simulink model "qcar_sensor_validation"  (R2024b)
settings: Solver=ode1  StartTime=0.0  StopTime=inf  FixedStep=Controller_Sample_Time  RelTol=1e-3  EnableMultiTasking=on
undefined symbols (not defined in the file): AAAF5050, angles_qcar2, cal_pos, Controller_Sample_Time, CSI_Sample_Time, gcbh, GyroKF_P0, GyroKF_Q, GyroKF_R, GyroKF_X0, height, HIL, ImageDisplay_Sample_Time, Initialization_Time, JPEG, K12, left, LiDAR_Sample_Time, MC, path_x4, path_y4, Point, qc_get_step_size, qcar2_lidar_to_body_rotation, qcar2_lidar_to_map_rotation, qcar2_virtual_to_physical_lidar_rotation, QCarEKF_L, QCarEKF_P0, QCarEKF_Q, QCarEKF_R_combined, QCarEKF_R_heading, QcarKF_X0, range_qcar2, RealSense_Sample_Time, steering_Kd, steering_Kp, top, video_display_show, width
libraries: quarc_library x45, simulink_extras x6, simulink x3, mspfiltlib x1
(part 2 of 3)

== system qcar_sensor_validation/writeToQCarDAC ==
  note: 11: LED left outside brake light
      | 12: LED left inside brake light
      | 12: LED right inside brake light
      | 13: LED right outside brake fight
      | 14: LED left reverse light
      | 15: LED right reverse light
      | 16: LED left rear signal
      | 17: LED right rear signal
      | 18: LED left outside headlight
      | 19: LED left middle headlight
      | 20: LED left inside headlight
      | 21: LED right inside headlight
      | 22: LED right middle headlight
      | 23: LED right outside headlight
      | 24: LED left front signal
      | 25: LED right front signal
  motor_cmd [1] (%) : Inport
  steering_cmd [1] (rad) : Inport  Port=2
  leds [14] (bool) : Inport  Port=3
  ledStrip [R,G,B] (%) : Inport  Port=4
  Gain : Gain
  HIL Write : quarc_library/Data Acquisition/Generic/Immediate I//O/HIL Write  object_name=HIL-2  analog_channels=[]  pwm_channels=[]  digital_channels=[11:26]  other_channels=[1000 11000]  sample_time=-1  active=on  vector_input=on
  LED Strip : quarc_library/Devices/Third-Party/Displays/LED Strip  led_type=AAAF5050-MC-K12  uri=tcpip://localhost:18969  mode=uniform  max_leds=33  initial_red=[0.000]  initial_green=[1.000]  initial_blue=[0.000]  final_red=[0]  final_green=[0]  final_blue=[0]  sample_time=ImageDisplay_Sample_Time  use_vectors=off  active=off
      settings: SourceProductName=QUARC Targets
  Mux : Mux  Inputs=2
  Steering Bias : Bias  Bias=-0.05  SaturateOnIntegerOverflow=off
  Terminator : Terminator
  motor sat : Saturate  UpperLimit=.6  LowerLimit=-0.6
  steering sat : Saturate
  wires:
  ledStrip [R,G,B] (%)/1 -> LED Strip/1
  steering_cmd [1] (rad)/1 -> Steering Bias/1
  motor sat/1 -> Mux/2
  steering sat/1 -> Mux/1
  leds [14] (bool)/1 -> HIL Write/1
  Steering Bias/1 -> Gain/1
  motor_cmd [1] (%)/1 -> motor sat/1
  LED Strip/1 -> Terminator/1
  Gain/1 -> steering sat/1
  Mux/1 -> HIL Write/2

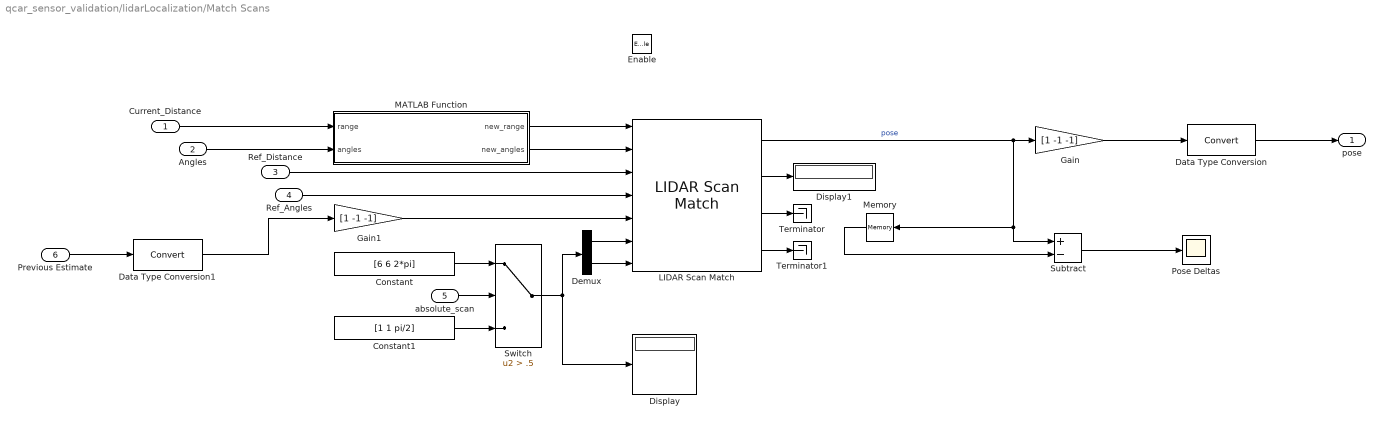
== system qcar_sensor_validation/lidarLocalization/Match Scans ==
  Current_Distance : Inport
  Angles : Inport  Port=2
  Ref_Distance : Inport  Port=3
  Ref_Angles : Inport  Port=4
  absolute_scan : Inport  Port=5
  Previous Estimate : Inport  Port=6
  Enable : EnablePort  PropagateVarSize=During execution
  Constant : Constant  Value=[6 6 2*pi]
  Constant1 : Constant  Value=[1 1 pi/2]
  Data Type Conversion : DataTypeConversion  SaturateOnIntegerOverflow=off  RndMeth=Floor
  Data Type Conversion1 : DataTypeConversion  SaturateOnIntegerOverflow=off  RndMeth=Floor
  Demux : Demux  Outputs=2
  Display : Display
  Display1 : Display
  Gain : Gain  Gain=[1 -1 -1]
  Gain1 : Gain  Gain=[1 -1 -1]
  LIDAR Scan Match : quarc_library/Image Processing/Generic/LIDAR Scan Match  mode=Variable-size input  resolution=35  max_range=8  use_initial_pose=on
      settings: SourceProductName=QUARC Targets
  MATLAB Function : MATLAB Function  TreatAsAtomicUnit=on
  Memory : Memory  InitialCondition=[0 0 0]  InheritSampleTime=on  LinearizeMemory=on  LinearizeAsDelay=on
  Pose Deltas : Scope
  Subtract : Sum  Inputs=+-
  Switch : Switch  Criteria=u2 > Threshold  Threshold=.5  SaturateOnIntegerOverflow=off  InputSameDT=off
  Terminator : Terminator
  Terminator1 : Terminator
  pose : Outport
  wires:
  LIDAR Scan Match/1 -> Subtract/1, Memory/1, Gain/1  "pose"
  Ref_Distance/1 -> LIDAR Scan Match/3
  Ref_Angles/1 -> LIDAR Scan Match/4
  Gain/1 -> Data Type Conversion/1
  Memory/1 -> Subtract/2
  absolute_scan/1 -> Switch/2
  Switch/1 -> Demux/1, Display/1
  Demux/1 -> LIDAR Scan Match/6
  Demux/2 -> LIDAR Scan Match/7
  Constant/1 -> Switch/1
  Constant1/1 -> Switch/3
  Data Type Conversion/1 -> pose/1
  MATLAB Function/1(new_range) -> LIDAR Scan Match/1
  MATLAB Function/2(new_angles) -> LIDAR Scan Match/2
  Subtract/1 -> Pose Deltas/1
  Previous Estimate/1 -> Data Type Conversion1/1
  Gain1/1 -> LIDAR Scan Match/5
  Data Type Conversion1/1 -> Gain1/1
  Current_Distance/1 -> MATLAB Function/1(range)
  Angles/1 -> MATLAB Function/2(angles)
  LIDAR Scan Match/3 -> Terminator/1
  LIDAR Scan Match/4 -> Terminator1/1
  LIDAR Scan Match/2 -> Display1/1

== system qcar_sensor_validation/lidarLocalization/RisingEdge ==
  Input : Inport
  Logical Operator1 : Logic  AllPortsSameDT=off
  Logical Operator2 : Logic  Operator=NOT  AllPortsSameDT=off
  Memory : Memory  InheritSampleTime=on  LinearizeMemory=on
  RisingEdgeTrigger : Outport  VectorParamsAs1DForOutWhenUnconnected=off
  wires:
  Logical Operator1/1 -> RisingEdgeTrigger/1
  Logical Operator2/1 -> Logical Operator1/2
  Memory/1 -> Logical Operator2/1
  Input/1 -> Logical Operator1/1, Memory/1

== system qcar_sensor_validation/lidarLocalization/rising edge latch ==
  rising edge trigger : Inport
  input : Inport  Port=2
  untriggered output : Inport  Port=3
  Latch Input : Subsystem  TreatAsAtomicUnit=on
  Switch : Switch  Threshold=0.5  SaturateOnIntegerOverflow=off  InputSameDT=off
  output : Outport  VectorParamsAs1DForOutWhenUnconnected=off
  wires:
  untriggered output/1 -> Switch/3
  Switch/1 -> output/1
  Latch Input/1(Latch) -> Switch/1
  Latch Input/2(Executed) -> Switch/2
  input/1 -> Latch Input/1(Input)
  rising edge trigger/1 -> Latch Input/Trigger

== system qcar_sensor_validation/obstacleDetection/Newer Depth ==
  In1 : Inport
  Channel : quarc_library/Signal Routing/Channel  channel=0  buffer_size=1
  Image Compress : quarc_library/Image Processing/Generic/Image Compress  algorithm=JPEG  source=Internal dialog parameter  quality=quality  output_dim=-1
  Video Display : quarc_library/Multimedia/Video Display  Tag=qcar_sensor_validation/obstacleDetection/Newer Depth/Video Display  sample_time=sample_time  use_hardware=on
  wires:
  Image Compress/1 -> Channel/1
  In1/1 -> Image Compress/1
  Channel/1 -> Video Display/1

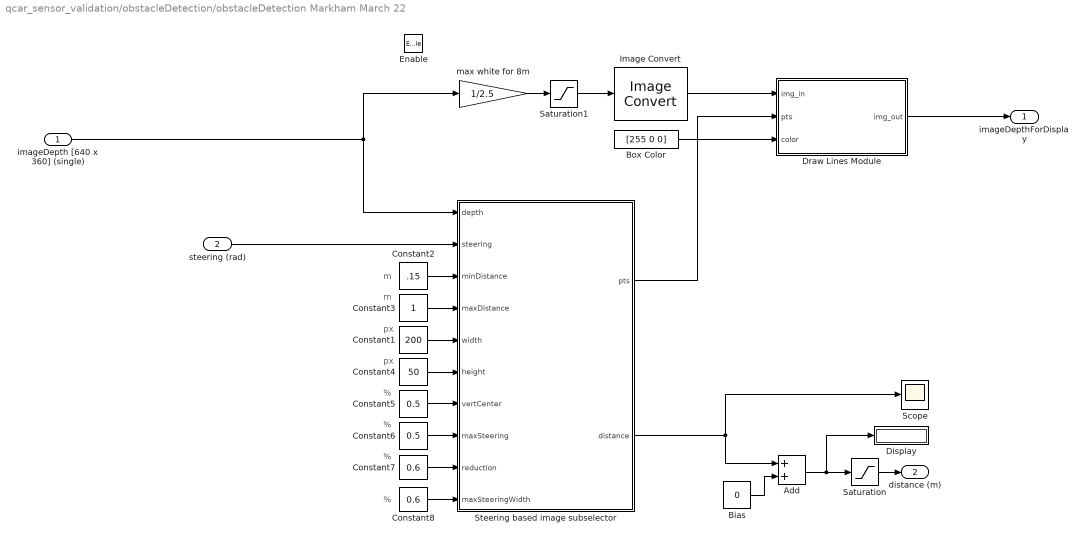
== system qcar_sensor_validation/obstacleDetection/obstacleDetection Markham March 22 ==
  note: %
  note: m
  note: m
  note: %
  note: px
  note: px
  note: %
  note: %
  imageDepth [640 x 360] (single) : Inport
  steering (rad) : Inport  Port=2
  Enable : EnablePort  PropagateVarSize=During execution
  Add : Sum
  Bias : Constant  Value=0
  Box Color : Constant  Value=[255 0 0]
  Constant1 : Constant  Value=200
  Constant2 : Constant  Value=.15
  Constant3 : Constant
  Constant4 : Constant  Value=50
  Constant5 : Constant  Value=0.5
  Constant6 : Constant  Value=0.5
  Constant7 : Constant  Value=0.6
  Constant8 : Constant  Value=0.6
  Display : Display
  Draw Lines Module : MATLAB Function  TreatAsAtomicUnit=on
  Image Convert : quarc_library/Image Processing/Generic/Image Convert  input_format=MATLAB greyscale (HxW)  padding=0  output_format=MATLAB greyscale (HxW)  data_type=uint16
      settings: AttributesFormatString=(%<input_format>)  SourceProductName=QUARC Targets
  Saturation : Saturate  UpperLimit=2  LowerLimit=0.05
  Saturation1 : Saturate  UpperLimit=1  LowerLimit=0
  Scope : Scope
  Steering based image subselector : MATLAB Function  TreatAsAtomicUnit=on
  max white for 8m : Gain  Gain=1/2.5
  imageDepthForDisplay : Outport  VectorParamsAs1DForOutWhenUnconnected=off
  distance (m) : Outport  Port=2  VectorParamsAs1DForOutWhenUnconnected=off
  wires:
  Saturation1/1 -> Image Convert/1
  Constant6/1 -> Steering based image subselector/8(maxSteering)
  Steering based image subselector/2(distance) -> Add/1, Scope/1
  Constant5/1 -> Steering based image subselector/7(vertCenter)
  Constant4/1 -> Steering based image subselector/6(height)
  Constant1/1 -> Steering based image subselector/5(width)
  Constant3/1 -> Steering based image subselector/4(maxDistance)
  Constant2/1 -> Steering based image subselector/3(minDistance)
  steering (rad)/1 -> Steering based image subselector/2(steering)
  Draw Lines Module/1(img_out) -> imageDepthForDisplay/1
  Steering based image subselector/1(pts) -> Draw Lines Module/2(pts)
  Image Convert/1 -> Draw Lines Module/1(img_in)
  max white for 8m/1 -> Saturation1/1
  imageDepth [640 x 360] (single)/1 -> Steering based image subselector/1(depth), max white for 8m/1
  Bias/1 -> Add/2
  Add/1 -> Saturation/1, Display/1
  Saturation/1 -> distance (m)/1
  Box Color/1 -> Draw Lines Module/3(color)
  Constant7/1 -> Steering based image subselector/9(reduction)
  Constant8/1 -> Steering based image subselector/10(maxSteeringWidth)

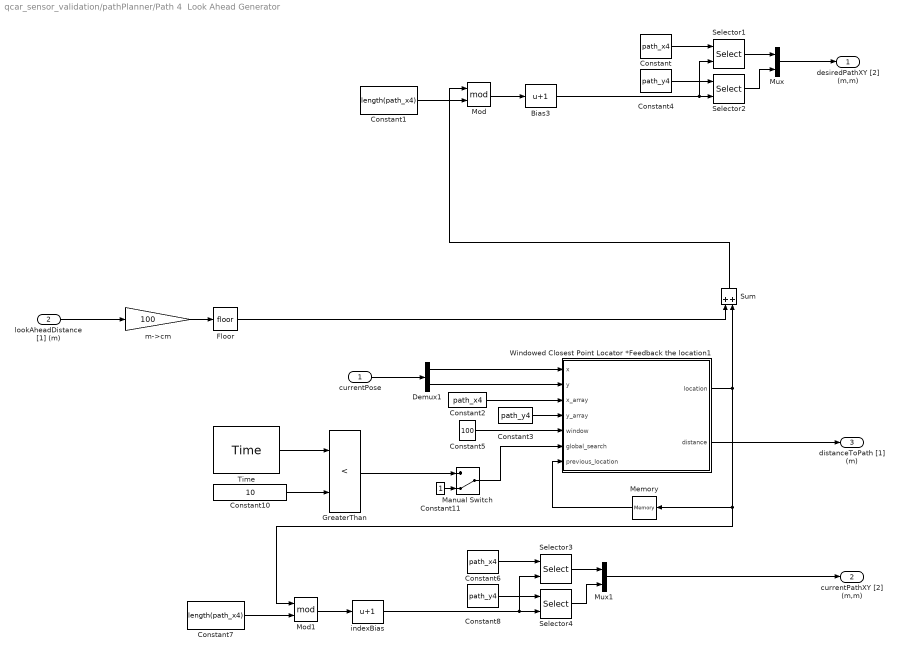
== system qcar_sensor_validation/pathPlanner/Path 4  Look Ahead Generator ==
  currentPose : Inport
  lookAheadDistance [1] (m) : Inport  Port=2
  Bias3 : Bias  Bias=1  SaturateOnIntegerOverflow=off
  Constant : Constant  Value=path_x4
  Constant1 : Constant  Value=length(path_x4)
  Constant10 : Constant  Value=10
  Constant11 : Constant
  Constant2 : Constant  Value=path_x4
  Constant3 : Constant  Value=path_y4
  Constant4 : Constant  Value=path_y4
  Constant5 : Constant  Value=100
  Constant6 : Constant  Value=path_x4
  Constant7 : Constant  Value=length(path_x4)
  Constant8 : Constant  Value=path_y4
  Demux1 : Demux  Outputs=2
  Floor : Rounding
  GreaterThan : RelationalOperator  Operator=<  OutDataTypeStr=boolean  RndMeth=Simplest  InputSameDT=off
  Manual Switch : ManualSwitch  CurrentSetting=0
  Memory : Memory  InitialCondition=1  InheritSampleTime=on  LinearizeMemory=on  LinearizeAsDelay=on
  Mod : Math  Operator=mod
  Mod1 : Math  Operator=mod
  Mux : Mux  Inputs=2
  Mux1 : Mux  Inputs=2
  Selector{1..4} (4 alike) : Selector  InputPortWidth=length(path_x4)  IndexOptions=Index vector (port)  Indices=[1 3]  OutputSizes=1
  Sum : Sum
  Time : quarc_library/Sources/Time/Time  time_source=Wall clock  sample_time=qc_get_step_size
  Windowed Closest Point Locator *Feedback the location1 : MATLAB Function  TreatAsAtomicUnit=on
  indexBias : Bias  Bias=1  SaturateOnIntegerOverflow=off
  m->cm : Gain  Gain=100
  desiredPathXY [2] (m,m) : Outport
  currentPathXY [2] (m,m) : Outport  Port=2
  distanceToPath [1] (m) : Outport  Port=3
  wires:
  Windowed Closest Point Locator *Feedback the location1/1(location) -> Mod1/1, Memory/1, Sum/2
  Memory/1 -> Windowed Closest Point Locator *Feedback the location1/7(previous_location)
  Constant5/1 -> Windowed Closest Point Locator *Feedback the location1/5(window)
  Bias3/1 -> Selector2/2, Selector1/2
  Windowed Closest Point Locator *Feedback the location1/2(distance) -> distanceToPath [1] (m)/1
  Selector2/1 -> Mux/2
  Mux/1 -> desiredPathXY [2] (m,m)/1
  Constant4/1 -> Selector2/1
  Selector1/1 -> Mux/1
  Constant/1 -> Selector1/1
  Floor/1 -> Sum/1
  m->cm/1 -> Floor/1
  lookAheadDistance [1] (m)/1 -> m->cm/1
  currentPose/1 -> Demux1/1
  Mod/1 -> Bias3/1
  Demux1/2 -> Windowed Closest Point Locator *Feedback the location1/2(y)
  Sum/1 -> Mod/1
  Constant1/1 -> Mod/2
  Constant3/1 -> Windowed Closest Point Locator *Feedback the location1/4(y_array)
  Constant2/1 -> Windowed Closest Point Locator *Feedback the location1/3(x_array)
  Demux1/1 -> Windowed Closest Point Locator *Feedback the location1/1(x)
  Mux1/1 -> currentPathXY [2] (m,m)/1
  Mod1/1 -> indexBias/1
  Selector4/1 -> Mux1/2
  Constant7/1 -> Mod1/2
  Selector3/1 -> Mux1/1
  Constant8/1 -> Selector4/1
  indexBias/1 -> Selector3/2, Selector4/2
  Constant6/1 -> Selector3/1
  Time/1 -> GreaterThan/1
  Constant10/1 -> GreaterThan/2
  Manual Switch/1 -> Windowed Closest Point Locator *Feedback the location1/6(global_search)
  Constant11/1 -> Manual Switch/2
  GreaterThan/1 -> Manual Switch/1

== system qcar_sensor_validation/pathPlanner/rateAligner ==
  xy 1 : Inport
  xy 2 : Inport  Port=2
  Demux1 : Demux  Outputs=2
  Demux2 : Demux  Outputs=2
  Mux : Mux  Inputs=2
  Mux1 : Mux  Inputs=2
  Rate Transition1 : RateTransition  OutPortSampleTime=ImageDisplay_Sample_Time
  Rate Transition2 : RateTransition  OutPortSampleTime=ImageDisplay_Sample_Time
  x : Outport
  y : Outport  Port=2
  wires:
  Demux2/1 -> Mux/2
  Demux1/2 -> Mux1/1
  Demux1/1 -> Mux/1
  Demux2/2 -> Mux1/2
  Mux/1 -> x/1
  Mux1/1 -> y/1
  xy 1/1 -> Rate Transition1/1
  Rate Transition1/1 -> Demux1/1
  xy 2/1 -> Rate Transition2/1
  Rate Transition2/1 -> Demux2/1

== system qcar_sensor_validation/rateTimingPlots/monitorTiming ==
  note: Timing Performance
  note: moniorTiming Module:
      |
      | This subsystem outputs the sample time and computation time of the model.
      |
      | Outputs:
      | sampleTime (s) n/a : Sample time (unfiltered and filtered) in seconds.
      | computationTime (s) n/a : Computation time (unfiltered and filtered) in seconds.
      |
      | Usage:
      | Compare the Sample Time (s) output to a constant (qc_get_step_size) to monitor whether or not the desired sample time is being achieved. The Computation Time (s) values should be lower than the corresponding sample time value to ensure that the solver has enough time per time step.
  Computation Time : quarc_library/Sources/Time/Computation Time  sample_time=CSI_Sample_Time  use_model=on  use_cpu_time=off
  Constant : Constant  Value=CSI_Sample_Time  SampleTime=-1
  Mux : Mux  Inputs=3
  Sample Time : quarc_library/Sources/Time/Sample Time  Priority=-99  sample_time=CSI_Sample_Time
  Timing (s) : Outport  VectorParamsAs1DForOutWhenUnconnected=off
  wires:
  Computation Time/1 -> Mux/3
  Mux/1 -> Timing (s)/1
  Sample Time/1 -> Mux/1
  Constant/1 -> Mux/2

== system qcar_sensor_validation/rateTimingPlots/monitorTiming1 ==
  note: moniorTiming Module:
      |
      | This subsystem outputs the sample time and computation time of the model.
      |
      | Outputs:
      | sampleTime (s) n/a : Sample time (unfiltered and filtered) in seconds.
      | computationTime (s) n/a : Computation time (unfiltered and filtered) in seconds.
      |
      | Usage:
      | Compare the Sample Time (s) output to a constant (qc_get_step_size) to monitor whether or not the desired sample time is being achieved. The Computation Time (s) values should be lower than the corresponding sample time value to ensure that the solver has enough time per time step.
  note: Timing Performance
  Computation Time : quarc_library/Sources/Time/Computation Time  sample_time=qc_get_step_size  use_model=on  use_cpu_time=off
  Constant : Constant  Value=qc_get_step_size  SampleTime=-1
  Mux : Mux  Inputs=3
  Sample Time : quarc_library/Sources/Time/Sample Time  Priority=-99  sample_time=qc_get_step_size
  Timing (s) : Outport  VectorParamsAs1DForOutWhenUnconnected=off
  wires:
  Constant/1 -> Mux/2
  Sample Time/1 -> Mux/1
  Mux/1 -> Timing (s)/1
  Computation Time/1 -> Mux/3

== system qcar_sensor_validation/rateTimingPlots/monitorTiming2 ==
  note: moniorTiming Module:
      |
      | This subsystem outputs the sample time and computation time of the model.
      |
      | Outputs:
      | sampleTime (s) n/a : Sample time (unfiltered and filtered) in seconds.
      | computationTime (s) n/a : Computation time (unfiltered and filtered) in seconds.
      |
      | Usage:
      | Compare the Sample Time (s) output to a constant (qc_get_step_size) to monitor whether or not the desired sample time is being achieved. The Computation Time (s) values should be lower than the corresponding sample time value to ensure that the solver has enough time per time step.
  note: Timing Performance
  Computation Time : quarc_library/Sources/Time/Computation Time  sample_time=RealSense_Sample_Time  use_model=on  use_cpu_time=off
  Constant : Constant  Value=RealSense_Sample_Time  SampleTime=-1
  Mux : Mux  Inputs=3
  Sample Time : quarc_library/Sources/Time/Sample Time  Priority=-99  sample_time=RealSense_Sample_Time
  Timing (s) : Outport  VectorParamsAs1DForOutWhenUnconnected=off
  wires:
  Constant/1 -> Mux/2
  Sample Time/1 -> Mux/1
  Mux/1 -> Timing (s)/1
  Computation Time/1 -> Mux/3

== system qcar_sensor_validation/rateTimingPlots/monitorTiming3 ==
  note: Timing Performance
  note: moniorTiming Module:
      |
      | This subsystem outputs the sample time and computation time of the model.
      |
      | Outputs:
      | sampleTime (s) n/a : Sample time (unfiltered and filtered) in seconds.
      | computationTime (s) n/a : Computation time (unfiltered and filtered) in seconds.
      |
      | Usage:
      | Compare the Sample Time (s) output to a constant (qc_get_step_size) to monitor whether or not the desired sample time is being achieved. The Computation Time (s) values should be lower than the corresponding sample time value to ensure that the solver has enough time per time step.
  Computation Time : quarc_library/Sources/Time/Computation Time  sample_time=ImageDisplay_Sample_Time  use_model=on  use_cpu_time=off
  Constant : Constant  Value=ImageDisplay_Sample_Time  SampleTime=-1
  Mux : Mux  Inputs=3
  Sample Time : quarc_library/Sources/Time/Sample Time  Priority=-99  sample_time=ImageDisplay_Sample_Time
  Timing (s) : Outport  VectorParamsAs1DForOutWhenUnconnected=off
  wires:
  Computation Time/1 -> Mux/3
  Mux/1 -> Timing (s)/1
  Sample Time/1 -> Mux/1
  Constant/1 -> Mux/2

== system qcar_sensor_validation/rateTimingPlots/monitorTiming5 ==
  note: moniorTiming Module:
      |
      | This subsystem outputs the sample time and computation time of the model.
      |
      | Outputs:
      | sampleTime (s) n/a : Sample time (unfiltered and filtered) in seconds.
      | computationTime (s) n/a : Computation time (unfiltered and filtered) in seconds.
      |
      | Usage:
      | Compare the Sample Time (s) output to a constant (qc_get_step_size) to monitor whether or not the desired sample time is being achieved. The Computation Time (s) values should be lower than the corresponding sample time value to ensure that the solver has enough time per time step.
  note: Timing Performance
  Computation Time : quarc_library/Sources/Time/Computation Time  sample_time=LiDAR_Sample_Time  use_model=on  use_cpu_time=off
  Constant : Constant  Value=LiDAR_Sample_Time  SampleTime=-1
  Mux : Mux  Inputs=3
  Sample Time : quarc_library/Sources/Time/Sample Time  Priority=-99  sample_time=LiDAR_Sample_Time
  Timing (s) : Outport  VectorParamsAs1DForOutWhenUnconnected=off
  wires:
  Constant/1 -> Mux/2
  Sample Time/1 -> Mux/1
  Mux/1 -> Timing (s)/1
  Computation Time/1 -> Mux/3

== system qcar_sensor_validation/rateTimingPlots/monitorTiming7 ==
  note: Timing Performance
  note: moniorTiming Module:
      |
      | This subsystem outputs the sample time and computation time of the model.
      |
      | Outputs:
      | sampleTime (s) n/a : Sample time (unfiltered and filtered) in seconds.
      | computationTime (s) n/a : Computation time (unfiltered and filtered) in seconds.
      |
      | Usage:
      | Compare the Sample Time (s) output to a constant (qc_get_step_size) to monitor whether or not the desired sample time is being achieved. The Computation Time (s) values should be lower than the corresponding sample time value to ensure that the solver has enough time per time step.
  Computation Time : quarc_library/Sources/Time/Computation Time  sample_time=1  use_model=on  use_cpu_time=off
  Constant : Constant  SampleTime=-1
  Mux : Mux  Inputs=3
  Sample Time : quarc_library/Sources/Time/Sample Time  Priority=-99  sample_time=1
  Timing (s) : Outport  VectorParamsAs1DForOutWhenUnconnected=off
  wires:
  Computation Time/1 -> Mux/3
  Mux/1 -> Timing (s)/1
  Sample Time/1 -> Mux/1
  Constant/1 -> Mux/2

== system qcar_sensor_validation/readQCarDAC/counts to meters ==
  note: Estimate car speed from motor encoder counts rate
  note: v = 2*pi*r * omega (if omega is in rot/s)
      | v = r * omega (if omega is in rad/s)
      | r = 0.0342 m
  note: (Diff. pinion*pinion)/(Spur*Diff. spur)
  note: speedEstimation Module:
      |
      | This subsystem converts the motor speed measurements in counts/s to a useful longitudinal car speed in m/s.
      |
      | Inputs:
      | motorSpeed (counts/s) n/a : Drive motor speed measured using an encoder
      |
      | Outputs:
      | longitudinalCarSpeed (m/s) n/a : The platform's longitudinal speed (along the front-rear axis direction)
  motorSpeed (counts/s) : Inport
  counts to rotations : Gain  Gain=1/720/4
  gear ratios : Gain  Gain=(13*19)/(70*37)
  rot/s to rad/s : Gain  Gain=2*pi
  wheel radius : Gain  Gain=0.0342
  longitudinalCarSpeed (m/s) : Outport  VectorParamsAs1DForOutWhenUnconnected=off
  wires:
  motorSpeed (counts/s)/1 -> counts to rotations/1
  rot/s to rad/s/1 -> wheel radius/1  "wheel speed (rad/s)"
  counts to rotations/1 -> gear ratios/1  "motor speed (rot/s)"
  wheel radius/1 -> longitudinalCarSpeed (m/s)/1  "wheel speed (m/s)"
  gear ratios/1 -> rot/s to rad/s/1  "shaft speed (rots/s)"

== system qcar_sensor_validation/readQCarDAC/counts//s to m//s ==
  note: speedEstimation Module:
      |
      | This subsystem converts the motor speed measurements in counts/s to a useful longitudinal car speed in m/s.
      |
      | Inputs:
      | motorSpeed (counts/s) n/a : Drive motor speed measured using an encoder
      |
      | Outputs:
      | longitudinalCarSpeed (m/s) n/a : The platform's longitudinal speed (along the front-rear axis direction)
  note: (Diff. pinion*pinion)/(Spur*Diff. spur)
  note: v = 2*pi*r * omega (if omega is in rot/s)
      | v = r * omega (if omega is in rad/s)
      | r = 0.0342 m
  note: Estimate car speed from motor encoder counts rate
  motorSpeed (counts/s) : Inport
  counts to rotations : Gain  Gain=1/720/4
  gear ratios : Gain  Gain=(13*19)/(70*37)
  rot/s to rad/s : Gain  Gain=2*pi
  wheel radius : Gain  Gain=0.0342
  longitudinalCarSpeed (m/s) : Outport  VectorParamsAs1DForOutWhenUnconnected=off
  wires:
  gear ratios/1 -> rot/s to rad/s/1  "shaft speed (rots/s)"
  wheel radius/1 -> longitudinalCarSpeed (m/s)/1  "wheel speed (m/s)"
  counts to rotations/1 -> gear ratios/1  "motor speed (rot/s)"
  rot/s to rad/s/1 -> wheel radius/1  "wheel speed (rad/s)"
  motorSpeed (counts/s)/1 -> counts to rotations/1

== system qcar_sensor_validation/readQCarDAC/powerConsumptionMonitor ==
  note: Battery percentage calculation
  note: P = VI
  note: Electrical
      | power
      | consumed
  note: Power Monitoring Module:
      |
      | This subsystem monitors power consumption and provides a percentage battery remaining indicator.
      |
      | Inputs:
      | motorCurrent (A) n/a : Motor current being pulled by the main drive motor
      | batteryVoltage (V) {0, 12.6} : Current battery voltage reading
      |
      | Outputs:
      | motorPowerConsumption (W) n/a : Current power in Watts being pulled by the main drive motor
      | batteryLevel (%) {0,1} : Percentage battery level remaining
      |
      | Usage:
      | This is based on a maximum 3S battery voltage of 12.6 V (4.2V per cell) and minimum of 10.5 V (3.5V per cell)
  motorCurrent (A) [1] : Inport
  batteryVoltage (V) [1] : Inport  Port=2
  Divide : Product  Inputs=*/
  Gain : Gain  Gain=100
  Product : Product
  Subtract : Sum  Inputs=+-
  Subtract1 : Sum  Inputs=+-
  max voltage : Constant  Value=12.6
  min voltage : Constant  Value=10.5
  motorPowerConsumption (W) [1] : Outport  VectorParamsAs1DForOutWhenUnconnected=off
  batteryLevel (%) [1] : Outport  Port=2  VectorParamsAs1DForOutWhenUnconnected=off
  wires:
  Divide/1 -> Gain/1
  Subtract1/1 -> Divide/2
  Gain/1 -> batteryLevel (%) [1]/1
  Product/1 -> motorPowerConsumption (W) [1]/1
  min voltage/1 -> Subtract/2, Subtract1/2
  motorCurrent (A) [1]/1 -> Product/1
  max voltage/1 -> Subtract1/1
  Subtract/1 -> Divide/1
  batteryVoltage (V) [1]/1 -> Subtract/1, Product/2

== system qcar_sensor_validation/speedController/realsenseObstacleDetectionSpeedAdjust ==
  obstacleDistance [1] (m) : Inport
  desiredSpeed [1] (m/s) : Inport  Port=2
  Constant : Constant  Value=0.375
  Constant2 : Constant  Value=0.6
  MATLAB Function : MATLAB Function  TreatAsAtomicUnit=on
  objectDetectionAdjustedSpeed [1] (m/s) : Outport  VectorParamsAs1DForOutWhenUnconnected=off
  wires:
  Constant2/1 -> MATLAB Function/3(nominal_tracking_distance)  "nominal tracking distance (m)"
  Constant/1 -> MATLAB Function/2(stop_distance)  "stop distance (m)"
  obstacleDistance [1] (m)/1 -> MATLAB Function/1(obstacle_distance)
  MATLAB Function/1(speed_cmd) -> objectDetectionAdjustedSpeed [1] (m/s)/1
  desiredSpeed [1] (m/s)/1 -> MATLAB Function/4(nominal_speed)

== system qcar_sensor_validation/speedController/speedController ==
  note: Feedforward
  note: Feedback
  arm [1] (bool) : Inport
  desiredSpeed (m/s) : Inport  Port=2
  currentSpeed (m/s) : Inport  Port=3
  Add : Sum
  Add1 : Sum
  Compare To Zero : simulink/Logic and Bit Operations/Compare To Zero  relop===  OutDataTypeStr=boolean
  Integrator1 : Integrator  ExternalReset=either  LimitOutput=on  UpperSaturationLimit=0.4  LowerSaturationLimit=-0.4
  Kff (% / m/s) : Gain  Gain=0.1
  "Ki (% / m) " : Gain
  Kp (% / m/s) : Gain  Gain=.3
  Multiply : Product
  Multiply1 : Product
  Multiply2 : Product
  Speed_Tracking : Scope  NumInputPorts=2
  Sum : Sum  Inputs=|+-
  command saturation : Saturate  UpperLimit=5  LowerLimit=-5
  throttleCmd (%) : Outport  VectorParamsAs1DForOutWhenUnconnected=off
  wires:
  command saturation/1 -> Multiply1/1  "desired"
  arm [1] (bool)/1 -> Multiply2/2, Multiply1/2, Multiply/2
  currentSpeed (m/s)/1 -> Multiply/1  "meas"
  Multiply/1 -> Sum/2, Speed_Tracking/2  "measured"
  Add/1 -> Add1/2
  Add1/1 -> Multiply2/1  "%"
  Multiply1/1 -> Compare To Zero/1, Sum/1, Kff (% / m/s)/1, Speed_Tracking/1  "desired"
  Integrator1/1 -> Add/2
  Kp (% / m/s)/1 -> Add/1
  Compare To Zero/1 -> Integrator1/2
  Kff (% / m/s)/1 -> Add1/1
  Sum/1 -> "Ki (% / m) "/1, Kp (% / m/s)/1
  "Ki (% / m) "/1 -> Integrator1/1
  Multiply2/1 -> throttleCmd (%)/1  "pwm duty cycle"
  desiredSpeed (m/s)/1 -> command saturation/1

== system qcar_sensor_validation/speedController/turnSpeedHandler ==
  speedCmd [1] (m/s) : Inport
  steeringCmd [1] (rad) : Inport  Port=2
  Cos ^ (attentuation) : Inport  Port=3
  Cos : Trigonometry  Operator=cos
  Product : Product
  Speed Comparison : Scope  NumInputPorts=2
  Square : Math  Operator=pow  SignedPower=on
  attenuationLimits : Saturate  UpperLimit=1  LowerLimit=.3
  attenuatedSpeedCmd [1] (m/s) : Outport  VectorParamsAs1DForOutWhenUnconnected=off
  wires:
  Cos/1 -> Square/1
  attenuationLimits/1 -> Product/2
  speedCmd [1] (m/s)/1 -> Product/1, Speed Comparison/1  "Input Speed"
  Cos ^ (attentuation)/1 -> Square/2
  Square/1 -> attenuationLimits/1
  Product/1 -> attenuatedSpeedCmd [1] (m/s)/1, Speed Comparison/2
  steeringCmd [1] (rad)/1 -> Cos/1  "input steering"

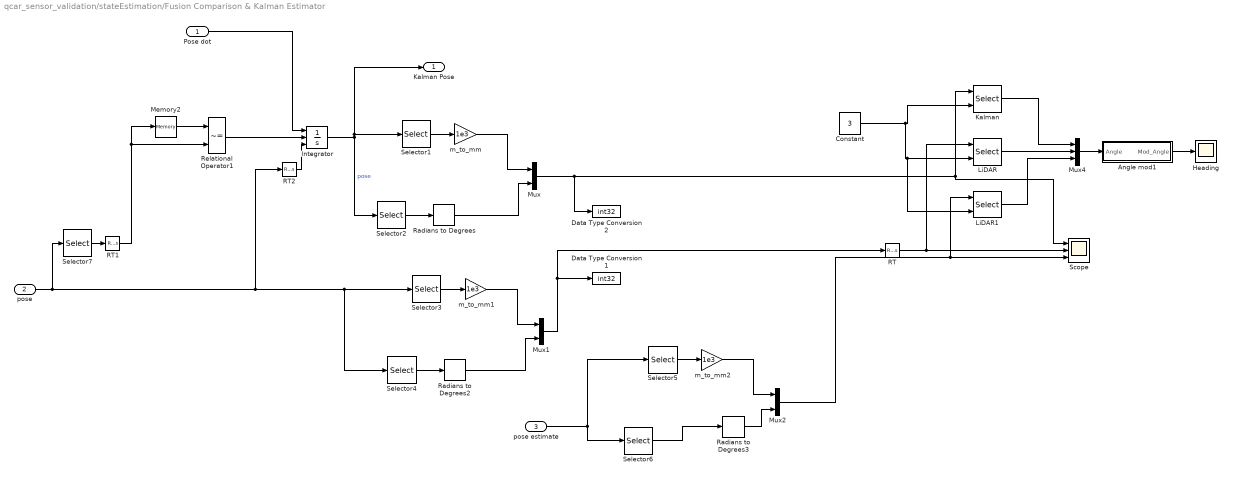
== system qcar_sensor_validation/stateEstimation/Fusion Comparison & Kalman Estimator ==
  Pose dot : Inport
  pose : Inport  Port=2
  pose estimate : Inport  Port=3
  Angle mod1 : Subsystem
  Constant : Constant  Value=3
  Data Type Conversion1 : DataTypeConversion  OutDataTypeStr=int32  RndMeth=Round  SaturateOnIntegerOverflow=off
  Data Type Conversion2 : DataTypeConversion  OutDataTypeStr=int32  RndMeth=Round  SaturateOnIntegerOverflow=off
  Heading : Scope
  Integrator : Integrator  ExternalReset=level  InitialConditionSource=external  WrappedStateUpperValue=[20 20 pi]  WrappedStateLowerValue=-[20 20 pi]
  Kalman : Selector  InputPortWidth=3  IndexOptions=Index vector (port)  Indices=[1 3]  OutputSizes=1
  LiDAR : Selector  InputPortWidth=3  IndexOptions=Index vector (port)  Indices=[1 3]  OutputSizes=1
  LiDAR1 : Selector  InputPortWidth=3  IndexOptions=Index vector (port)  Indices=[1 3]  OutputSizes=1
  Memory2 : Memory  InheritSampleTime=on  LinearizeMemory=on  LinearizeAsDelay=on
  Mux : Mux  Inputs=2
  Mux1 : Mux  Inputs=2
  Mux2 : Mux  Inputs=2
  Mux4 : Mux  Inputs=3
  RT : RateTransition  OutPortSampleTime=qc_get_step_size
  RT1 : RateTransition  OutPortSampleTime=qc_get_step_size
  RT2 : RateTransition  OutPortSampleTime=qc_get_step_size
  Radians to Degrees : simulink_extras/Transformations/Radians to Degrees
  Radians to Degrees2 : simulink_extras/Transformations/Radians to Degrees
  Radians to Degrees3 : simulink_extras/Transformations/Radians to Degrees
  Relational Operator1 : RelationalOperator  Operator=~=  OutDataTypeStr=boolean  RndMeth=Simplest  InputSameDT=off
  Scope : Scope  NumInputPorts=3
  Selector1 : Selector  InputPortWidth=3  IndexOptions=Index vector (dialog)  Indices=1:2  OutputSizes=1
  Selector2 : Selector  InputPortWidth=3  IndexOptions=Index vector (dialog)  Indices=3  OutputSizes=1
  Selector3 : Selector  InputPortWidth=3  IndexOptions=Index vector (dialog)  Indices=1:2  OutputSizes=1
  Selector4 : Selector  InputPortWidth=3  IndexOptions=Index vector (dialog)  Indices=3  OutputSizes=1
  Selector5 : Selector  InputPortWidth=3  IndexOptions=Index vector (dialog)  Indices=1:2  OutputSizes=1
  Selector6 : Selector  InputPortWidth=3  IndexOptions=Index vector (dialog)  Indices=3  OutputSizes=1
  Selector7 : Selector  InputPortWidth=3  IndexOptions=Index vector (dialog)  Indices=1  OutputSizes=1
  m_to_mm : Gain  Gain=1e3
  m_to_mm1 : Gain  Gain=1e3
  m_to_mm2 : Gain  Gain=1e3
  Kalman Pose : Outport
  wires:
  Mux2/1 -> LiDAR1/1, Scope/3
  Selector6/1 -> Radians to Degrees3/1
  m_to_mm2/1 -> Mux2/1
  Integrator/1 -> Kalman Pose/1, Selector1/1, Selector2/1  "pose"
  Selector1/1 -> m_to_mm/1
  pose estimate/1 -> Selector6/1, Selector5/1
  Selector5/1 -> m_to_mm2/1
  Selector4/1 -> Radians to Degrees2/1
  Radians to Degrees3/1 -> Mux2/2
  Mux/1 -> Scope/1, Kalman/1, Data Type Conversion2/1
  m_to_mm1/1 -> Mux1/1
  Selector2/1 -> Radians to Degrees/1
  Pose dot/1 -> Integrator/1
  m_to_mm/1 -> Mux/1
  Mux1/1 -> Data Type Conversion1/1, RT/1
  Radians to Degrees/1 -> Mux/2
  Selector3/1 -> m_to_mm1/1
  Radians to Degrees2/1 -> Mux1/2
  RT/1 -> LiDAR/1, Scope/2
  pose/1 -> Selector7/1, Selector4/1, Selector3/1, RT2/1
  RT2/1 -> Integrator/3
  RT1/1 -> Memory2/1, Relational Operator1/2
  Memory2/1 -> Relational Operator1/1
  Selector7/1 -> RT1/1
  Relational Operator1/1 -> Integrator/2
  Mux4/1 -> Angle mod1/1(Angle)
  LiDAR/1 -> Mux4/2
  Kalman/1 -> Mux4/1
  LiDAR1/1 -> Mux4/3
  Constant/1 -> LiDAR1/2, LiDAR/2, Kalman/2
  Angle mod1/1(Mod_Angle) -> Heading/1

== system qcar_sensor_validation/stateEstimation/Gyro KF + EKF ==
  speed : Inport
  delta : Inport  Port=2
  x_gps : Inport  Port=3
  y_gps : Inport  Port=4
  th_gps : Inport  Port=5
  thd_gyro : Inport  Port=6
  newGPSData : Inport  Port=7
  Heading Kalman Filter : MATLAB Function  TreatAsAtomicUnit=on
  QCar EKF : MATLAB Function  TreatAsAtomicUnit=on
  Xhat : Outport
  gyro_bias : Outport  Port=2
  wires:
  x_gps/1 -> QCar EKF/3(x_gps)
  y_gps/1 -> QCar EKF/4(y_gps)
  Heading Kalman Filter/1(th_hat) -> QCar EKF/5(th_hat)
  newGPSData/1 -> QCar EKF/6(newGPSData), Heading Kalman Filter/3(newGPSData)
  delta/1 -> QCar EKF/2(delta)
  thd_gyro/1 -> Heading Kalman Filter/1(thd_gyro)
  speed/1 -> QCar EKF/1(speed)
  QCar EKF/1(Xhat) -> Xhat/1
  th_gps/1 -> Heading Kalman Filter/2(th_gps)
  Heading Kalman Filter/2(gyro_bias) -> gyro_bias/1

== system qcar_sensor_validation/stateEstimation/Sensor Fusion - Complementary Filter ==
  note: One idead is to have the integrator reset if rate is high...
  note: stable gains Kp = 0.4*.4
  car speed : Inport
  rate : Inport  Port=2
  correction : Inport  Port=3
  Constant : Constant
  Constant1 : Constant  Value=5
  Constant2 : Constant  Value=.1
  Correction_Weight : Scope
  Display : Display
  Gain : Gain  Gain=[100 100 1]
  Integrator : Integrator  WrappedStateUpperValue=[20 20 pi]  WrappedStateLowerValue=-[20 20 pi]
  Integrator1 : Integrator  ExternalReset=level  LimitOutput=on  UpperSaturationLimit=.05*[1 1 1]*1  LowerSaturationLimit=-.05*[1 1 1]*1
  MATLAB Function : MATLAB Function  TreatAsAtomicUnit=on
  Manual Switch : ManualSwitch  CurrentSetting=0
  Product : Product
  Scope : Scope  NumInputPorts=2
  Subtract : Sum  Inputs=+-
  Subtract1 : Sum  Inputs=+-
  Subtract2 : Sum
  ki : Gain  Gain=[4 4 4]*1
  kp : Gain  Gain=[1 1 1]*.400*1
  estimate : Outport  VectorParamsAs1DForOutWhenUnconnected=off
  wires:
  Integrator/1 -> Subtract/1, estimate/1
  Subtract/1 -> ki/1, kp/1
  Integrator1/1 -> Scope/1, Subtract2/2
  kp/1 -> Scope/2, Subtract2/1
  Subtract1/1 -> Integrator/1
  ki/1 -> Integrator1/1
  correction/1 -> Subtract/2
  rate/1 -> Subtract1/1
  Manual Switch/1 -> Integrator1/2
  Constant/1 -> Manual Switch/1
  car speed/1 -> MATLAB Function/1(car_speed)
  MATLAB Function/1(correction_weight) -> Correction_Weight/1, Product/1, Display/1
  Subtract2/1 -> Gain/1
  Product/1 -> Subtract1/2
  Constant1/1 -> MATLAB Function/2(slope)
  Constant2/1 -> MATLAB Function/3(min_weight)
  Gain/1 -> Product/2

== system qcar_sensor_validation/stateEstimation/Subsystem ==
  Angle : Inport
  Bias : Bias  Bias=pi  SaturateOnIntegerOverflow=off
  Bias1 : Bias  Bias=-pi  SaturateOnIntegerOverflow=off
  Constant1 : Constant  Value=2*pi
  Mod : Math  Operator=mod
  Mod_Angle : Outport
  wires:
  Mod/1 -> Bias1/1
  Constant1/1 -> Mod/2
  Bias/1 -> Mod/1
  Bias1/1 -> Mod_Angle/1
  Angle/1 -> Bias/1

== system qcar_sensor_validation/stateEstimation/Subsystem1 ==
  Angle : Inport
  Bias : Bias  Bias=pi  SaturateOnIntegerOverflow=off
  Bias1 : Bias  Bias=-pi  SaturateOnIntegerOverflow=off
  Constant1 : Constant  Value=2*pi
  Mod : Math  Operator=mod
  Mod_Angle : Outport
  wires:
  Angle/1 -> Bias/1
  Bias1/1 -> Mod_Angle/1
  Bias/1 -> Mod/1
  Constant1/1 -> Mod/2
  Mod/1 -> Bias1/1

== system qcar_sensor_validation/stateEstimation/bicycleModel ==
  note: coordinate transformation
  note: Model side slip angle beta
  note: steering servo dynamics
  heading (rad) : Inport
  steering [1] (rad) : Inport  Port=2
  carSpeed (m/s) : Inport  Port=3
  z_gyroscope (rad/s) : Inport  Port=4
  Add : Sum
  Divide : Product  Inputs=*/
  Lr : Constant  Value=0.128
  Mux3 : Mux  Inputs=3
  Product : Product
  Product1 : Product
  Product2 : Product
  Transfer Fcn : TransferFcn  Denominator=[0.1026 1]
  Trigonometric Function : Trigonometry
  Trigonometric Function1 : Trigonometry  Operator=cos
  Trigonometric Function2 : Trigonometry  Operator=tan
  Trigonometric Function3 : Trigonometry  Operator=atan
  steering servo dynamics : Scope  NumInputPorts=2
  wheelbase : Constant  Value=0.256
  "poseRate (m/s, m/s, rad/s)" : Outport  VectorParamsAs1DForOutWhenUnconnected=off
  wires:
  Add/1 -> Trigonometric Function1/1, Trigonometric Function/1
  Trigonometric Function1/1 -> Product1/2
  Product/1 -> Mux3/2  "y_dot"
  steering [1] (rad)/1 -> Transfer Fcn/1, steering servo dynamics/1  "delta"
  carSpeed (m/s)/1 -> Product/2, Product1/1  "v"
  Product1/1 -> Mux3/1  "x_dot"
  Trigonometric Function/1 -> Product/1
  z_gyroscope (rad/s)/1 -> Mux3/3  "psi_dot"
  heading (rad)/1 -> Add/1  "psi"
  Mux3/1 -> "poseRate (m/s, m/s, rad/s)"/1
  Transfer Fcn/1 -> Trigonometric Function2/1, steering servo dynamics/2
  Divide/1 -> Trigonometric Function3/1
  wheelbase/1 -> Divide/2
  Product2/1 -> Divide/1  "Lr tan(delta)"
  Trigonometric Function3/1 -> Add/2  "beta"
  Trigonometric Function2/1 -> Product2/1  "tan(delta)"
  Lr/1 -> Product2/2  "Lr"

== system qcar_sensor_validation/stateEstimation/xy signal maker ==
  xy 1 : Inport
  xy 2 : Inport  Port=2
  Demux1 : Demux  Outputs=2
  Demux2 : Demux  Outputs=2
  Mux : Mux  Inputs=2
  Mux1 : Mux  Inputs=2
  Rate Transition1 : RateTransition  OutPortSampleTime=ImageDisplay_Sample_Time
  Rate Transition2 : RateTransition  OutPortSampleTime=ImageDisplay_Sample_Time
  x : Outport
  y : Outport  Port=2
  wires:
  Demux2/1 -> Mux/2
  Demux1/2 -> Mux1/1
  Demux1/1 -> Mux/1
  Demux2/2 -> Mux1/2
  Mux/1 -> x/1
  Mux1/1 -> y/1
  xy 1/1 -> Rate Transition1/1
  Rate Transition1/1 -> Demux1/1
  xy 2/1 -> Rate Transition2/1
  Rate Transition2/1 -> Demux2/1

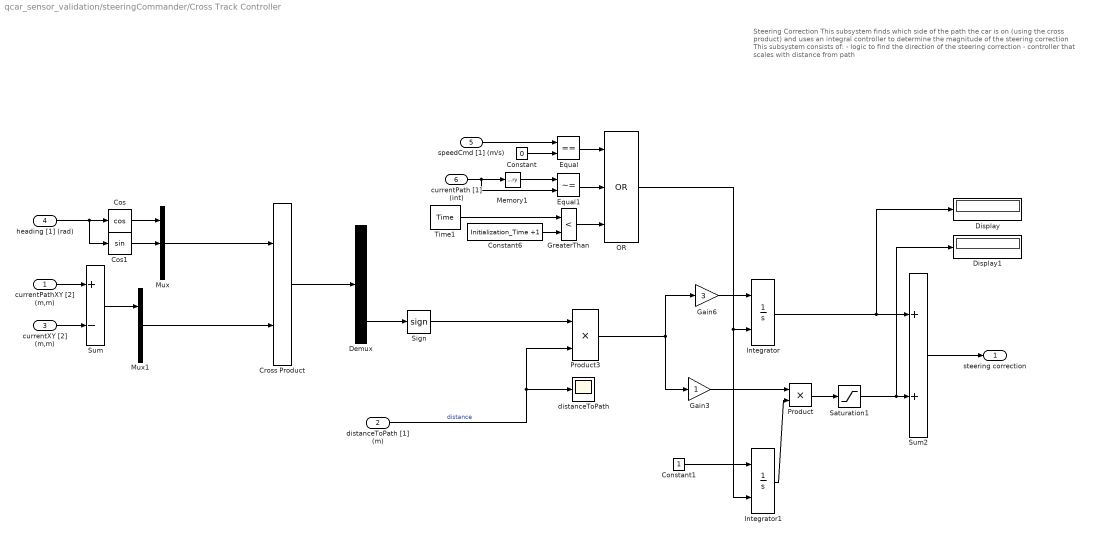
== system qcar_sensor_validation/steeringCommander/Cross Track Controller ==
  note: Steering Correction
      |
      | This subsystem finds which side of the path the car is on (using the cross product) and uses an integral controller to determine the magnitude of the steering correction
      |
      | This subsystem consists of:
      |
      | - logic to find the direction of the steering correction
      | - controller that scales with distance from path
  currentPathXY [2] (m,m) : Inport
  distanceToPath [1] (m) : Inport  Port=2
  currentXY [2] (m,m) : Inport  Port=3
  heading [1] (rad) : Inport  Port=4
  speedCmd [1] (m/s) : Inport  Port=5
  currentPath [1] (int) : Inport  Port=6
  Constant : Constant  Value=0
  Constant1 : Constant
  Constant6 : Constant  Value=Initialization_Time +1
  Cos : Trigonometry  Operator=cos
  Cos1 : Trigonometry
  Cross Product : quarc_library/Math Operations/Vectors/Cross Product
      settings: SourceProductName=QUARC Targets
  Demux : Demux  Outputs=3
  Display : Display
  Display1 : Display
  Equal : RelationalOperator  Operator===  OutDataTypeStr=boolean  RndMeth=Simplest  InputSameDT=off
  Equal1 : RelationalOperator  Operator=~=  OutDataTypeStr=boolean  RndMeth=Simplest  InputSameDT=off
  Gain3 : Gain
  Gain6 : Gain  Gain=3
  GreaterThan : RelationalOperator  Operator=<  OutDataTypeStr=boolean  RndMeth=Simplest  InputSameDT=off
  Integrator : Integrator  ExternalReset=level  LimitOutput=on  UpperSaturationLimit=.2  LowerSaturationLimit=-.2
  Integrator1 : Integrator  ExternalReset=level  LimitOutput=on  UpperSaturationLimit=1  LowerSaturationLimit=0
  Memory1 : Memory  InitialCondition=6  InheritSampleTime=on  LinearizeMemory=on  LinearizeAsDelay=on
  Mux : Mux  Inputs=3
  Mux1 : Mux  Inputs=2
  OR : Logic  Operator=OR  Inputs=3  IconShape=distinctive  AllPortsSameDT=off  OutDataTypeStr=boolean
  Product : Product
  Product3 : Product
  Saturation1 : Saturate  UpperLimit=.2  LowerLimit=-.2
  Sign : Signum
  Sum : Sum  Inputs=+-
  Sum2 : Sum
  Time1 : quarc_library/Sources/Time/Time  time_source=Wall clock  sample_time=qc_get_step_size
  distanceToPath : Scope
  steering correction : Outport
  wires:
  heading [1] (rad)/1 -> Cos1/1, Cos/1
  Cos/1 -> Mux/1
  Cos1/1 -> Mux/2
  currentXY [2] (m,m)/1 -> Sum/2
  currentPathXY [2] (m,m)/1 -> Sum/1
  Sum/1 -> Mux1/1
  Mux1/1 -> Cross Product/2
  Mux/1 -> Cross Product/1
  Cross Product/1 -> Demux/1
  Demux/3 -> Sign/1
  Sign/1 -> Product3/1
  Gain6/1 -> Integrator/1
  Product3/1 -> Gain3/1, Gain6/1
  Integrator/1 -> Display/1, Sum2/1
  Saturation1/1 -> Display1/1, Sum2/2
  distanceToPath [1] (m)/1 -> Product3/2, distanceToPath/1  "distance"
  Sum2/1 -> steering correction/1
  speedCmd [1] (m/s)/1 -> Equal/1
  Constant/1 -> Equal/2
  currentPath [1] (int)/1 -> Equal1/2, Memory1/1
  Memory1/1 -> Equal1/1
  Equal1/1 -> OR/2
  Equal/1 -> OR/1
  OR/1 -> Integrator1/2, Integrator/2
  Constant1/1 -> Integrator1/1
  Product/1 -> Saturation1/1
  Gain3/1 -> Product/1
  Integrator1/1 -> Product/2
  Time1/1 -> GreaterThan/1
  Constant6/1 -> GreaterThan/2
  GreaterThan/1 -> OR/3

== system qcar_sensor_validation/steeringCommander/Steering Based on LiDAR ==
  yawRate [1] (rad/s) : Inport
  xy_desired [2] (m,m) : Inport  Port=2
  xy [2] (m,m) : Inport  Port=3
  heading [1] (rad) : Inport  Port=4
  Enable : EnablePort  PropagateVarSize=During execution
  D : Gain  Gain=steering_Kd
  Demux : Demux  Outputs=2
  Gyro Filter : TransferFcn  Numerator=[25]  Denominator=[1 25]
  If : If  IfExpression=u1 < -pi  ElseIfExpressions=u1 > pi
  If Action Subsystem : Subsystem  TreatAsAtomicUnit=on
  If Action Subsystem1 : Subsystem  TreatAsAtomicUnit=on
  If Action Subsystem2 : Subsystem  TreatAsAtomicUnit=on
  Merge : Merge  Inputs=3
  P : Gain  Gain=steering_Kp
  Sum : Sum  Inputs=+-
  Sum1 : Sum  Inputs=|+-
  Sum3 : Sum  Inputs=+-
  Trigonometric Function : Trigonometry  Operator=atan2
  lidarSteering [1] (rad) : Outport
  wires:
  If/1 -> If Action Subsystem/Action
  If/2 -> If Action Subsystem1/Action
  If/3 -> If Action Subsystem2/Action
  Sum3/1 -> If Action Subsystem1/1(aoa [1] (rad)), If Action Subsystem/1(aoa [1] (rad)), If Action Subsystem2/1(aoa [1] (rad)), If/1  "steering_angle"
  If Action Subsystem/1(steering [1] (rad)) -> Merge/1
  If Action Subsystem1/1(steering [1] (rad)) -> Merge/2
  If Action Subsystem2/1(steering [1] (rad)) -> Merge/3
  Demux/1 -> Trigonometric Function/2
  xy [2] (m,m)/1 -> Sum/2
  xy_desired [2] (m,m)/1 -> Sum/1
  heading [1] (rad)/1 -> Sum3/2  "heading"
  Sum/1 -> Demux/1
  Demux/2 -> Trigonometric Function/1
  Merge/1 -> P/1  "wrapped output"
  D/1 -> Sum1/2  "poseRateCorrection"
  Sum1/1 -> lidarSteering [1] (rad)/1
  P/1 -> Sum1/1
  Trigonometric Function/1 -> Sum3/1  "heading"
  yawRate [1] (rad/s)/1 -> Gyro Filter/1  "poseRate"
  Gyro Filter/1 -> D/1  "yaw rate"

== system qcar_sensor_validation/lidarLocalization/rising edge latch/Latch Input ==
  Input : Inport
  Trigger : TriggerPort  VariantControl=(inherit)
  Constant : Constant
  Latch : Outport  VectorParamsAs1DForOutWhenUnconnected=off
  Executed : Outport  Port=2  VectorParamsAs1DForOutWhenUnconnected=off
  wires:
  Constant/1 -> Executed/1
  Input/1 -> Latch/1

== system qcar_sensor_validation/stateEstimation/Fusion Comparison & Kalman Estimator/Angle mod1 ==
  Angle : Inport
  Bias : Bias  Bias=180  SaturateOnIntegerOverflow=off
  Bias1 : Bias  Bias=-180  SaturateOnIntegerOverflow=off
  Constant1 : Constant  Value=360
  Mod : Math  Operator=mod
  Mod_Angle : Outport
  wires:
  Angle/1 -> Bias/1
  Bias1/1 -> Mod_Angle/1
  Bias/1 -> Mod/1
  Constant1/1 -> Mod/2
  Mod/1 -> Bias1/1

== system qcar_sensor_validation/steeringCommander/Steering Based on LiDAR/If Action Subsystem ==
  aoa [1] (rad) : Inport
  Action Port : ActionPort  ActionPortLabel=if(u1 < -pi)
  Bias : Bias  Bias=2*pi  SaturateOnIntegerOverflow=off
  steering [1] (rad) : Outport
  wires:
  aoa [1] (rad)/1 -> Bias/1
  Bias/1 -> steering [1] (rad)/1

== system qcar_sensor_validation/steeringCommander/Steering Based on LiDAR/If Action Subsystem1 ==
  aoa [1] (rad) : Inport
  Action Port : ActionPort  ActionPortLabel=elseif(u1 > pi)
  Bias : Bias  Bias=-2*pi  SaturateOnIntegerOverflow=off
  steering [1] (rad) : Outport
  wires:
  Bias/1 -> steering [1] (rad)/1
  aoa [1] (rad)/1 -> Bias/1

== system qcar_sensor_validation/steeringCommander/Steering Based on LiDAR/If Action Subsystem2 ==
  aoa [1] (rad) : Inport
  Action Port : ActionPort  ActionPortLabel=else
  Bias : Bias  SaturateOnIntegerOverflow=off
  steering [1] (rad) : Outport
  wires:
  aoa [1] (rad)/1 -> Bias/1
  Bias/1 -> steering [1] (rad)/1

== matlab function qcar_sensor_validation/stateEstimation/Gyro KF + EKF/Heading Kalman Filter ==
  settings: updateMethod=DISCRETE
  data: thd_gyro input; th_gps input; newGPSData input; GyroKF_Q parameter; GyroKF_R parameter; GyroKF_X0 parameter; GyroKF_P0 parameter; th_hat output; gyro_bias output; Controller_Sample_Time parameter
function [th_hat, gyro_bias] = GyroKF(thd_gyro, th_gps, newGPSData, GyroKF_Q, GyroKF_R, GyroKF_X0, GyroKF_P0, Controller_Sample_Time)

    persistent X_hat P I A B C
    if isempty(X_hat)
        % State and Covarience estimates
        X_hat = GyroKF_X0;
        P = GyroKF_P0;

        % Statespace model matrices
        I = eye(2);
        A = I + Controller_Sample_Time*[0, -1;
                                   0, 0];
        B = Controller_Sample_Time*[1;
                               0];
        C = [1, 0];
    end

    % Prediction
    X_hat = A*X_hat + B*thd_gyro;
    P = A*P*A' + GyroKF_Q;

    % Correction 
    if newGPSData
        P_times_CTransposed = P*C';
        S = C*P_times_CTransposed + GyroKF_R;
        K = P_times_CTransposed / S;

        z = wrapToPi(th_gps - C*X_hat);

        X_hat = X_hat + K*z;
        X_hat(1) = wrapToPi(X_hat(1));

        P = (I - K*C) * P;
    end
    
    th_hat = X_hat(1);
    gyro_bias = X_hat(2);
end

== matlab function qcar_sensor_validation/stateEstimation/Gyro KF + EKF/QCar EKF ==
  settings: updateMethod=DISCRETE
  data: speed input; delta input; x_gps input; Xhat output; y_gps input; th_hat input; newGPSData input; Controller_Sample_Time parameter; QCarEKF_P0 parameter; QcarKF_X0 parameter; QCarEKF_R_heading parameter; QCarEKF_Q parameter; QCarEKF_L parameter; QCarEKF_R_combined parameter
function Xhat  = QCarEKF(speed, delta, x_gps, y_gps, th_hat, newGPSData, Controller_Sample_Time, QCarEKF_P0, QcarKF_X0, QCarEKF_R_heading, QCarEKF_Q, QCarEKF_L, QCarEKF_R_combined)




    persistent X_hat P I C_heading C_combined
    if isempty(X_hat)
        % State and Covarience estimates
        X_hat = QcarKF_X0;
        P = QCarEKF_P0;

        % Statespace model matrices
        I = eye(3);
        
        C_heading = [0, 0, 1];
        C_combined = eye(3);
    end
    
    dt = Controller_Sample_Time;
    x = X_hat(1);
    y = X_hat(2);
    th = X_hat(3);
    
    % Prediction:
    F = [1, 0, -dt*speed*sin(th);
         0, 1,  dt*speed*cos(th);
         0, 0,             1];
    P = F*P*F' + QCarEKF_Q;
    
    X_hat = X_hat + dt*speed * [cos(th);
                            sin(th);
                            tan(delta) / QCarEKF_L];
                         
    
    % Correction
    if newGPSData
        y = [x_gps; y_gps; th_hat];
        C = C_combined;
        R = QCarEKF_R_combined;
        
    else
        y = th_hat;
        C = C_heading;
        R = QCarEKF_R_heading;
    end

    P_times_CTransposed = P*C';
    S = C*P_times_CTransposed + R;
    K = P_times_CTransposed / S;

    z = y - C*X_hat;
    if newGPSData
        z(3) = wrapToPi(z(3));
    else
        z = wrapToPi(z);
    end

    X_hat = X_hat + K*z;
    X_hat(3) = wrapToPi(X_hat(3));

    P = (I - K*C) * P;
    
    Xhat = X_hat;
end

== matlab function qcar_sensor_validation/lidarLocalization/Match Scans/MATLAB Function ==
  data: new_range output size=SPR_qcar2 [..SPR_qcar2]; range input [1..SPR_qcar2]; angles input [1..SPR_qcar2]; new_angles output size=SPR_qcar2 [..SPR_qcar2]
function [new_range, new_angles]  = clean_zero_readings(range, angles)
range_indicies = find (range == 0);
range(range_indicies) = [];
angles(range_indicies) = [];
new_range = range;
new_angles = angles;
end

== matlab function qcar_sensor_validation/quat2eul ==
  data: q input; yaw output
function yaw = quat2yaw(q)
% q : 1x4 quaternion [w x y z]

% Crear quaternion
qq = quaternion(q(1), q(2), q(3), q(4));

% Convertir a Euler (rad), ZYX = yaw-pitch-roll
eul = euler(qq, "ZYX", "frame");

% Extraer yaw (Z)
yaw = eul(1);

== matlab function qcar_sensor_validation/pathPlanner/Path 4  Look Ahead Generator/Windowed Closest Point Locator *Feedback the location1 ==
  data: x input; location output; y input; x_array input; y_array input; window input; global_search input; distance output; previous_location input
function [location,distance] = find_closest_window_point(x,y,x_array,y_array, window, global_search, previous_location)
distance = 1e6;
location = previous_location;
array_length = length (x_array);

if (global_search == 1)
    
    %Search the whole array (usually at startup)
    for i =1:array_length
        d = (x-x_array(i))^2 + (y-y_array(i))^2;
        if d < distance
            distance = d;
            location = i;
        end
    end
    
else
    
    if (location + window) > array_length
        %We need to wrap from the end
        % loop one - end of array:
        for i = (location-window):array_length
            d = (x-x_array(i))^2 + (y-y_array(i))^2;
            if d < distance
                distance = d;
                location = i;
            end
        end
        % loop two - start of array:
        for i = 1:(location+window-array_length)
            d = (x-x_array(i))^2 + (y-y_array(i))^2;
            if d < distance
                distance = d;
                location = i;
            end
        end
        
    elseif (location-window) < 1
        %We need to wrap from the beginning
        % loop one - end of array:
        for i = (array_length+location-window):array_length
            d = (x-x_array(i))^2 + (y-y_array(i))^2;
            if d < distance
                distance = d;
                location = i;
            end
        end
        % loop two - start of array:
        for i = 1:(location+window)
            d = (x-x_array(i))^2 + (y-y_array(i))^2;
            if d < distance
                distance = d;
                location = i;
            end
        end
        
    else
        %no need to wrap
        for i = (location-window):(location+window)
            d = (x-x_array(i))^2 + (y-y_array(i))^2;
            if d < distance
                distance = d;
                location = i;
            end
        end
    end
    
end
distance = sqrt(distance);
end

== matlab function qcar_sensor_validation/Normalize Depth ==
  data: depth input; out output
function out = normalizeDepth(depth)

dmin = min(depth(:));
dmax = max(depth(:));

out = (depth - dmin) / (dmax - dmin);

end

== matlab function qcar_sensor_validation/stateEstimation/Sensor Fusion - Complementary Filter/MATLAB Function ==
  data: car_speed input; correction_weight output; slope input; min_weight input
function correction_weight = weighting(car_speed, slope, min_weight)
correction_weight = 1 - 1*slope*car_speed;
if correction_weight < min_weight
    correction_weight = min_weight;
end
end

== matlab function qcar_sensor_validation/speedController/realsenseObstacleDetectionSpeedAdjust/MATLAB Function ==
  data: obstacle_distance input; speed_cmd output; stop_distance input; nominal_tracking_distance input; nominal_speed input
function speed_cmd = adaptive_cruise_control(obstacle_distance, stop_distance, nominal_tracking_distance, nominal_speed)

speed_cmd = nominal_speed;

if obstacle_distance < stop_distance
    speed_cmd = sat(nominal_speed,0,-1);
    
elseif obstacle_distance < nominal_tracking_distance
    speed_cmd = nominal_speed/(nominal_tracking_distance-stop_distance)*obstacle_distance...
        - nominal_speed/(nominal_tracking_distance-stop_distance)*stop_distance;
    
end

function output = sat (input, max,min)
if input > max
    output = max;
elseif input < min
    output = min;
else
    output = input;
end
